simulink model "Model2_2023b"  (R2023b)
settings: Solver=ode4  StartTime=0.0  StopTime=100  FixedStep=0.01  RelTol=1e-3
values from neighbouring files (symbols this model uses):
  ARM_P_PID = [10 0 20]*0.1    [Single_ARM_Monte.m]    (also in main_starter.m)
  ARM_T_PID = [100 0 0]    [Single_ARM_Monte.m]    (also in main_starter.m)
  ARM_V_PID = [10 0 5]*0.1    [Single_ARM_Monte.m]    (also in main_starter.m)
  D_Joint0_angle0 = 45    [Single_ARM_Monte.m]    (also in main_starter.m)
  D_Joint0_angle1 = 0    [Single_ARM_Monte.m]    (also in main_starter.m)
  D_Joint0_angle2 = 0    [Single_ARM_Monte.m]    (also in main_starter.m)
  D_Joint0_rate0 = 0    [Single_ARM_Monte.m]    (also in main_starter.m)
  D_Joint0_rate1 = 0    [Single_ARM_Monte.m]    (also in main_starter.m)
  D_Joint0_rate2 = 0    [Single_ARM_Monte.m]    (also in main_starter.m)
  Joint_Motor_Mass = 23    [Single_ARM_Monte.m]    (also in main_starter.m)
  L_Joint0_angle0 = 45    [Single_ARM_Monte.m]    (also in main_starter.m)
  L_Joint0_angle1 = 0    [Single_ARM_Monte.m]    (also in main_starter.m)
  L_Joint0_angle2 = 0    [Single_ARM_Monte.m]    (also in main_starter.m)
  L_Joint0_rate0 = 0    [Single_ARM_Monte.m]    (also in main_starter.m)
  L_Joint0_rate1 = 0    [Single_ARM_Monte.m]    (also in main_starter.m)
  L_Joint0_rate2 = 0    [Single_ARM_Monte.m]    (also in main_starter.m)
  L_Joint_Offset = [ ... (first row only)    [Single_ARM_Monte.m]    (also in main_starter.m)
  Link1_Mass = 11    [Single_ARM_Monte.m]    (also in main_starter.m)
  Link2_Mass = 15.6    [Single_ARM_Monte.m]    (also in main_starter.m)
  Link3_Mass = 11    [Single_ARM_Monte.m]    (also in main_starter.m)
  Motor_transfer_Den = [1 100]    [Single_ARM_Monte.m]    (also in main_starter.m)
  Motor_transfer_Num = [100]    [Single_ARM_Monte.m]    (also in main_starter.m)
  PID_dt = 0.01    [Single_ARM_Monte.m]    (also in main_starter.m)
  R_Joint0_angle0 = 45    [Single_ARM_Monte.m]    (also in main_starter.m)
  R_Joint0_angle1 = 0    [Single_ARM_Monte.m]    (also in main_starter.m)
  R_Joint0_angle2 = 0    [Single_ARM_Monte.m]    (also in main_starter.m)
  R_Joint0_rate0 = 0    [Single_ARM_Monte.m]    (also in main_starter.m)
  R_Joint0_rate1 = 0    [Single_ARM_Monte.m]    (also in main_starter.m)
  R_Joint0_rate2 = 0    [Single_ARM_Monte.m]    (also in main_starter.m)
  RW_Att_D = 0.5    [Single_ARM_Monte.m]    (also in main_starter.m)
  RW_Att_I = 0.2    [Single_ARM_Monte.m]    (also in main_starter.m)
  RW_Att_P = 0.1    [Single_ARM_Monte.m]    (also in main_starter.m)
  RW_Mass = 100    [Single_ARM_Monte.m]    (also in main_starter.m)
  S_Body_Mass = 5    [Single_ARM_Monte.m]    (also in main_starter.m)
  S_init_pos = [0 0 0]'    [Single_ARM_Monte.m]    (also in main_starter.m)
  S_init_vel = [0 0 0]'    [Single_ARM_Monte.m]    (also in main_starter.m)
  T_Body_Mass = 4    [Single_ARM_Monte.m]    (also in main_starter.m)
  T_init_pos = [T_init_pos_list(i,1) T_init_pos_list(i,2) 0]'    [Single_ARM_Monte.m]    (also in main_starter.m = [1 0 0]')
  T_init_vel = [0 0 0]'    [Single_ARM_Monte.m]    (also in main_starter.m)
  Torq_mea_transfer_Den = [1 5]    [Single_ARM_Monte.m]    (also in main_starter.m)
  Torq_mea_transfer_Num = [5]    [Single_ARM_Monte.m]    (also in main_starter.m)
  U_Joint0_angle0 = 45    [Single_ARM_Monte.m]    (also in main_starter.m)
  U_Joint0_angle1 = 0    [Single_ARM_Monte.m]    (also in main_starter.m)
  U_Joint0_angle2 = 0    [Single_ARM_Monte.m]    (also in main_starter.m)
  U_Joint0_rate0 = 0    [Single_ARM_Monte.m]    (also in main_starter.m)
  U_Joint0_rate1 = 0    [Single_ARM_Monte.m]    (also in main_starter.m)
  U_Joint0_rate2 = 0    [Single_ARM_Monte.m]    (also in main_starter.m)
undefined symbols (not defined in the file or in its folder): X, Y, Z
libraries: nesl_utility x315, sm_lib x282, simulink_extras x46, sharedtransform x25, aerolibutil x4, simulink x2, matrix_library x2, dspmtrx3 x1
(part 1 of 12)
settings Model: Creator=yhj2019  LastModifiedBy=uscl
settings ExplorerConfigSet: InternalSimMechanicsExplorerSettings="<ExplorerConfiguration><canonicalview>default</canonicalview><AnimationSetting><BasePlaybackSpeed>1.0</BasePlaybackSpeed><PlaybackSpeedFactor>1.0</PlaybackSpeedFactor></AnimationSetting><TilePanel><TileInfo><Tiles Columns=\"1\" Count=\"1\" Rows=\"1\"><Column Weight=\"1\"/><Row Weight=\"1\"/><Tile Height=\"1\" Width=\"1\" X=\"0\" Y=\"0\"/></Tiles></TileInfo><SceneInfo><SceneViewer><BGColor><R>1</R><G>1</G><B>1</B></BGColor><Camera><DoPerspective>off</DoPerspective><Position><X>0.13582852589406158</X><Y>0.0815359438413352511</Y><Z>11.3316555905426526</Z></Position><Center><X>0.13582852589406158</X><Y>0.0815359438413352511</Y><Z>-0.00499986008405706173</Z></Center><Up><X>0</X><Y>1</Y><Z>-0</Z></Up><ViewLimDist>1</ViewLimDist><YLim>0.485687177104648538</YLim><XLim>0.453052070342676139</XLim></Camera></SceneViewer></SceneInfo></TilePanel><MechEditorPanel><Cameras/><GfxPanelCameraMap/><VideoCreator><PlaybackSpeedRatio>1.0</PlaybackSpeedRatio><FrameRate>30</FrameRate><VideoFormat>Motion JPEG AVI</VideoFormat><FrameSize>auto</FrameSize></VideoCreator></MechEditorPanel></ExplorerConfiguration>"

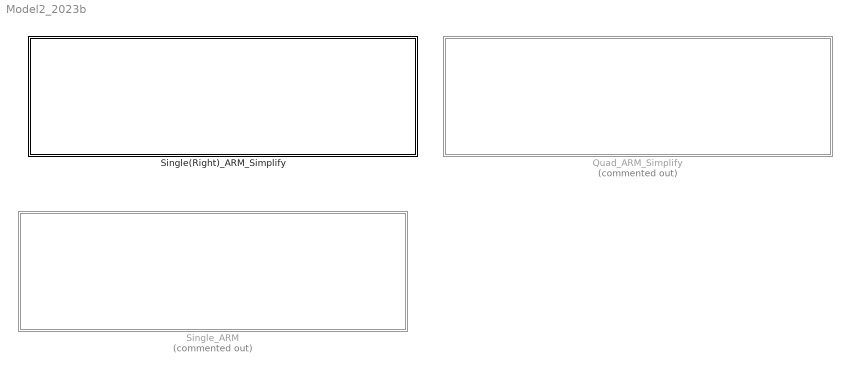
== system Model2_2023b ==
  Quad_ARM_Simplify : Subsystem  Commented=on
  Single(Right)_ARM_Simplify : Subsystem
  Single_ARM : Subsystem  Commented=on

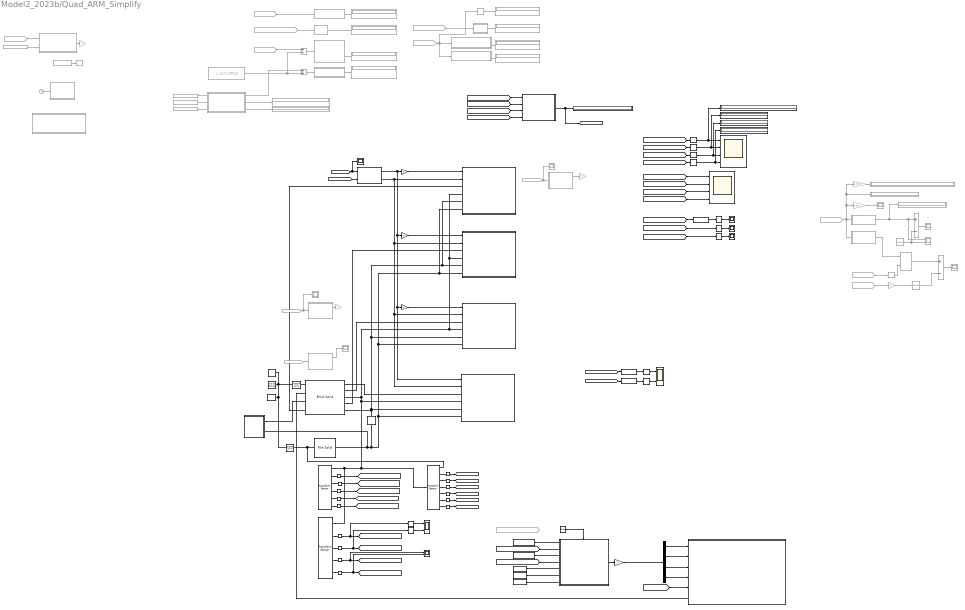
== system Model2_2023b/Quad_ARM_Simplify ==
  6-DOF Joint1 : sm_lib/Joints/6-DOF Joint  JointMode=Normal  CompositeWrenchDir=FollowerOnBase  CompositeWrenchFrame=BaseFrame  SenseConstraintForce=off  SenseConstraintTorque=off  SenseTotalForce=off  SenseTotalTorque=off  PxPositionTargetSpecify=on  PxPositionTargetPriority=High  PxPositionTargetValue=T_init_pos(1)  PxPositionTargetValueUnits=m  PxVelocityTargetSpecify=on  PxVelocityTargetPriority=High  PxVelocityTargetValue=T_init_vel(1)  PxVelocityTargetValueUnits=m/s  PxEquilibriumPosition=0  PxEquilibriumPositionUnits=m  PxSpringStiffness=0  PxSpringStiffnessUnits=N/m  PxDampingCoefficient=0  PxDampingCoefficientUnits=N/(m/s)  PxLowerLimitSpecify=off  PxLowerLimitBound=-1  PxLowerLimitBoundUnits=m  PxLowerLimitStiffness=1e6  PxLowerLimitStiffnessUnits=N/m  PxLowerLimitDamping=1e3  PxLowerLimitDampingUnits=N/(m/s)  PxLowerLimitTransitionRegionWidth=1e-4  PxLowerLimitTransitionRegionWidthUnits=m  PxUpperLimitSpecify=off  PxUpperLimitBound=1  PxUpperLimitBoundUnits=m  PxUpperLimitStiffness=1e6  PxUpperLimitStiffnessUnits=N/m  PxUpperLimitDamping=1e3  PxUpperLimitDampingUnits=N/(m/s)  PxUpperLimitTransitionRegionWidth=1e-4  PxUpperLimitTransitionRegionWidthUnits=m  PxTorqueActuationMode=NoTorque  PxMotionActuationMode=ComputedMotion  PxSensePosition=off  PxSenseVelocity=off  PxSenseAcceleration=off  PxSenseTorqueForce=off  PxSenseLowerLimitTorqueForce=off  PxSenseUpperLimitTorqueForce=off  PyPositionTargetSpecify=on  PyPositionTargetPriority=High  PyPositionTargetValue=T_init_pos(2)  PyPositionTargetValueUnits=m  PyVelocityTargetSpecify=on  PyVelocityTargetPriority=High  PyVelocityTargetValue=T_init_vel(2)  PyVelocityTargetValueUnits=m/s  PyEquilibriumPosition=0  PyEquilibriumPositionUnits=m  PySpringStiffness=0  PySpringStiffnessUnits=N/m  PyDampingCoefficient=0  PyDampingCoefficientUnits=N/(m/s)  PyLowerLimitSpecify=off  PyLowerLimitBound=-1  PyLowerLimitBoundUnits=m  PyLowerLimitStiffness=1e6  PyLowerLimitStiffnessUnits=N/m  PyLowerLimitDamping=1e3  PyLowerLimitDampingUnits=N/(m/s)  PyLowerLimitTransitionRegionWidth=1e-4  PyLowerLimitTransitionRegionWidthUnits=m  PyUpperLimitSpecify=off  PyUpperLimitBound=1  PyUpperLimitBoundUnits=m  PyUpperLimitStiffness=1e6  PyUpperLimitStiffnessUnits=N/m  PyUpperLimitDamping=1e3  PyUpperLimitDampingUnits=N/(m/s)  PyUpperLimitTransitionRegionWidth=1e-4  PyUpperLimitTransitionRegionWidthUnits=m  PyTorqueActuationMode=NoTorque  PyMotionActuationMode=ComputedMotion  PySensePosition=off  PySenseVelocity=off  PySenseAcceleration=off  PySenseTorqueForce=off  PySenseLowerLimitTorqueForce=off  PySenseUpperLimitTorqueForce=off  PzPositionTargetSpecify=on  PzPositionTargetPriority=High  PzPositionTargetValue=T_init_pos(3)  PzPositionTargetValueUnits=m  PzVelocityTargetSpecify=on  PzVelocityTargetPriority=High  PzVelocityTargetValue=T_init_vel(3)  PzVelocityTargetValueUnits=m/s  PzEquilibriumPosition=0  PzEquilibriumPositionUnits=m  PzSpringStiffness=0  PzSpringStiffnessUnits=N/m  PzDampingCoefficient=0  PzDampingCoefficientUnits=N/(m/s)  PzLowerLimitSpecify=off  PzLowerLimitBound=-1  PzLowerLimitBoundUnits=m  PzLowerLimitStiffness=1e6  PzLowerLimitStiffnessUnits=N/m  PzLowerLimitDamping=1e3  PzLowerLimitDampingUnits=N/(m/s)  PzLowerLimitTransitionRegionWidth=1e-4  PzLowerLimitTransitionRegionWidthUnits=m  PzUpperLimitSpecify=off  PzUpperLimitBound=1  PzUpperLimitBoundUnits=m  PzUpperLimitStiffness=1e6  PzUpperLimitStiffnessUnits=N/m  PzUpperLimitDamping=1e3  PzUpperLimitDampingUnits=N/(m/s)  PzUpperLimitTransitionRegionWidth=1e-4  PzUpperLimitTransitionRegionWidthUnits=m  PzTorqueActuationMode=NoTorque  PzMotionActuationMode=ComputedMotion  PzSensePosition=off  PzSenseVelocity=off  PzSenseAcceleration=off  PzSenseTorqueForce=off  PzSenseLowerLimitTorqueForce=off  PzSenseUpperLimitTorqueForce=off  SphPositionTargetSpecify=on  SphPositionTargetPriority=High  SphPositionTargetRotationMethod=RotationSequence  SphPositionTargetFollAlignAxisA=+X  SphPositionTargetBaseAlignAxisA=+Y  SphPositionTargetFollAlignAxisB=+Y  SphPositionTargetBaseAlignAxisB=+Z  SphPositionTargetRotationStandardAxis=+Z  SphPositionTargetRotationAngle=0.0  SphPositionTargetRotationAngleUnits=deg  SphPositionTargetRotationArbitraryAxis=[0 0 1]  SphPositionTargetRotationSequenceAxes=FollowerAxes  SphPositionTargetRotationSequence=ZYX  SphPositionTargetRotationSequenceAngles=T_init_att  SphPositionTargetRotationSequenceAnglesUnits=deg  SphPositionTargetRotationMatrix=[1 0 0; 0 1 0; 0 0 1]  SphPositionTargetQuaternion=[1 0 0 0]  SphVelocityTargetSpecify=on  SphVelocityTargetPriority=High  SphVelocityTargetValue=T_init_rate  SphVelocityTargetValueUnits=deg/s  SphVelocityTargetInFollowerFrame=on  SphEqPosRotationMethod=None  SphEqPosFollAlignAxisA=+X  SphEqPosBaseAlignAxisA=+Y  SphEqPosFollAlignAxisB=+Y  SphEqPosBaseAlignAxisB=+Z  SphEqPosRotationStandardAxis=+Z  SphEqPosRotationAngle=0.0  SphEqPosRotationAngleUnits=deg  SphEqPosRotationArbitraryAxis=[0 0 1]  SphEqPosRotationSequenceAxes=FollowerAxes  SphEqPosRotationSequence=XYX  SphEqPosRotationSequenceAngles=[0 0 0]  SphEqPosRotationSequenceAnglesUnits=deg  SphEqPosRotationMatrix=[1 0 0; 0 1 0; 0 0 1]  SphEqPosQuaternion=[1 0 0 0]  SphSpringStiffness=0  SphSpringStiffnessUnits=N*m/deg  SphDampingCoefficient=0  SphDampingCoefficientUnits=N*m/(deg/s)  SphLowerLimitSpecify=off  SphLowerLimitBound=15  SphLowerLimitBoundUnits=deg  SphLowerLimitStiffness=1e4  SphLowerLimitStiffnessUnits=N*m/deg  SphLowerLimitDamping=10  SphLowerLimitDampingUnits=N*m/(deg/s)  SphLowerLimitTransitionRegionWidth=0.1  SphLowerLimitTransitionRegionWidthUnits=deg  SphUpperLimitSpecify=off  SphUpperLimitBound=45  SphUpperLimitBoundUnits=deg  SphUpperLimitStiffness=1e4  SphUpperLimitStiffnessUnits=N*m/deg  SphUpperLimitDamping=10  SphUpperLimitDampingUnits=N*m/(deg/s)  SphUpperLimitTransitionRegionWidth=0.1  SphUpperLimitTransitionRegionWidthUnits=deg  SphTorqueActuationMode=NoTorque  SphActuateTorqueX=off  SphActuateTorqueY=off  SphActuateTorqueZ=off  SphActuateTorque=off  SphActuationFrame=BaseFrame  SphSensePosition=off  SphSenseVelocityX=off  SphSenseVelocityY=off  SphSenseVelocityZ=off  SphSenseVelocity=off  SphSenseAccelerationX=off  SphSenseAccelerationY=off  SphSenseAccelerationZ=off  SphSenseAcceleration=off  SphSenseLowerLimitTorqueMag=off  SphSenseUpperLimitTorqueMag=off  SphSensingFrame=BaseFrame
  6-DOF Joint2 : sm_lib/Joints/6-DOF Joint  JointMode=Normal  CompositeWrenchDir=FollowerOnBase  CompositeWrenchFrame=BaseFrame  SenseConstraintForce=off  SenseConstraintTorque=off  SenseTotalForce=off  SenseTotalTorque=off  PxPositionTargetSpecify=on  PxPositionTargetPriority=High  PxPositionTargetValue=S_init_pos(1)  PxPositionTargetValueUnits=m  PxVelocityTargetSpecify=on  PxVelocityTargetPriority=High  PxVelocityTargetValue=S_init_vel(1)  PxVelocityTargetValueUnits=m/s  PxEquilibriumPosition=0  PxEquilibriumPositionUnits=m  PxSpringStiffness=0  PxSpringStiffnessUnits=N/m  PxDampingCoefficient=0  PxDampingCoefficientUnits=N/(m/s)  PxLowerLimitSpecify=off  PxLowerLimitBound=-1  PxLowerLimitBoundUnits=m  PxLowerLimitStiffness=1e6  PxLowerLimitStiffnessUnits=N/m  PxLowerLimitDamping=1e3  PxLowerLimitDampingUnits=N/(m/s)  PxLowerLimitTransitionRegionWidth=1e-4  PxLowerLimitTransitionRegionWidthUnits=m  PxUpperLimitSpecify=off  PxUpperLimitBound=1  PxUpperLimitBoundUnits=m  PxUpperLimitStiffness=1e6  PxUpperLimitStiffnessUnits=N/m  PxUpperLimitDamping=1e3  PxUpperLimitDampingUnits=N/(m/s)  PxUpperLimitTransitionRegionWidth=1e-4  PxUpperLimitTransitionRegionWidthUnits=m  PxTorqueActuationMode=NoTorque  PxMotionActuationMode=ComputedMotion  PxSensePosition=off  PxSenseVelocity=off  PxSenseAcceleration=off  PxSenseTorqueForce=off  PxSenseLowerLimitTorqueForce=off  PxSenseUpperLimitTorqueForce=off  PyPositionTargetSpecify=on  PyPositionTargetPriority=High  PyPositionTargetValue=S_init_pos(2)  PyPositionTargetValueUnits=m  PyVelocityTargetSpecify=on  PyVelocityTargetPriority=High  PyVelocityTargetValue=S_init_vel(2)  PyVelocityTargetValueUnits=m/s  PyEquilibriumPosition=0  PyEquilibriumPositionUnits=m  PySpringStiffness=0  PySpringStiffnessUnits=N/m  PyDampingCoefficient=0  PyDampingCoefficientUnits=N/(m/s)  PyLowerLimitSpecify=off  PyLowerLimitBound=-1  PyLowerLimitBoundUnits=m  PyLowerLimitStiffness=1e6  PyLowerLimitStiffnessUnits=N/m  PyLowerLimitDamping=1e3  PyLowerLimitDampingUnits=N/(m/s)  PyLowerLimitTransitionRegionWidth=1e-4  PyLowerLimitTransitionRegionWidthUnits=m  PyUpperLimitSpecify=off  PyUpperLimitBound=1  PyUpperLimitBoundUnits=m  PyUpperLimitStiffness=1e6  PyUpperLimitStiffnessUnits=N/m  PyUpperLimitDamping=1e3  PyUpperLimitDampingUnits=N/(m/s)  PyUpperLimitTransitionRegionWidth=1e-4  PyUpperLimitTransitionRegionWidthUnits=m  PyTorqueActuationMode=NoTorque  PyMotionActuationMode=ComputedMotion  PySensePosition=off  PySenseVelocity=off  PySenseAcceleration=off  PySenseTorqueForce=off  PySenseLowerLimitTorqueForce=off  PySenseUpperLimitTorqueForce=off  PzPositionTargetSpecify=on  PzPositionTargetPriority=High  PzPositionTargetValue=S_init_pos(3)  PzPositionTargetValueUnits=m  PzVelocityTargetSpecify=on  PzVelocityTargetPriority=High  PzVelocityTargetValue=S_init_vel(3)  PzVelocityTargetValueUnits=m/s  PzEquilibriumPosition=0  PzEquilibriumPositionUnits=m  PzSpringStiffness=0  PzSpringStiffnessUnits=N/m  PzDampingCoefficient=0  PzDampingCoefficientUnits=N/(m/s)  PzLowerLimitSpecify=off  PzLowerLimitBound=-1  PzLowerLimitBoundUnits=m  PzLowerLimitStiffness=1e6  PzLowerLimitStiffnessUnits=N/m  PzLowerLimitDamping=1e3  PzLowerLimitDampingUnits=N/(m/s)  PzLowerLimitTransitionRegionWidth=1e-4  PzLowerLimitTransitionRegionWidthUnits=m  PzUpperLimitSpecify=off  PzUpperLimitBound=1  PzUpperLimitBoundUnits=m  PzUpperLimitStiffness=1e6  PzUpperLimitStiffnessUnits=N/m  PzUpperLimitDamping=1e3  PzUpperLimitDampingUnits=N/(m/s)  PzUpperLimitTransitionRegionWidth=1e-4  PzUpperLimitTransitionRegionWidthUnits=m  PzTorqueActuationMode=NoTorque  PzMotionActuationMode=ComputedMotion  PzSensePosition=off  PzSenseVelocity=off  PzSenseAcceleration=off  PzSenseTorqueForce=off  PzSenseLowerLimitTorqueForce=off  PzSenseUpperLimitTorqueForce=off  SphPositionTargetSpecify=on  SphPositionTargetPriority=High  SphPositionTargetRotationMethod=RotationSequence  SphPositionTargetFollAlignAxisA=+X  SphPositionTargetBaseAlignAxisA=+Y  SphPositionTargetFollAlignAxisB=+Y  SphPositionTargetBaseAlignAxisB=+Z  SphPositionTargetRotationStandardAxis=+Z  SphPositionTargetRotationAngle=0.0  SphPositionTargetRotationAngleUnits=deg  SphPositionTargetRotationArbitraryAxis=[0 0 1]  SphPositionTargetRotationSequenceAxes=FollowerAxes  SphPositionTargetRotationSequence=ZYX  SphPositionTargetRotationSequenceAngles=S_init_att  SphPositionTargetRotationSequenceAnglesUnits=deg  SphPositionTargetRotationMatrix=[1 0 0; 0 1 0; 0 0 1]  SphPositionTargetQuaternion=[1 0 0 0]  SphVelocityTargetSpecify=on  SphVelocityTargetPriority=High  SphVelocityTargetValue=S_init_rate  SphVelocityTargetValueUnits=deg/s  SphVelocityTargetInFollowerFrame=on  SphEqPosRotationMethod=None  SphEqPosFollAlignAxisA=+X  SphEqPosBaseAlignAxisA=+Y  SphEqPosFollAlignAxisB=+Y  SphEqPosBaseAlignAxisB=+Z  SphEqPosRotationStandardAxis=+Z  SphEqPosRotationAngle=0.0  SphEqPosRotationAngleUnits=deg  SphEqPosRotationArbitraryAxis=[0 0 1]  SphEqPosRotationSequenceAxes=FollowerAxes  SphEqPosRotationSequence=XYX  SphEqPosRotationSequenceAngles=[0 0 0]  SphEqPosRotationSequenceAnglesUnits=deg  SphEqPosRotationMatrix=[1 0 0; 0 1 0; 0 0 1]  SphEqPosQuaternion=[1 0 0 0]  SphSpringStiffness=0  SphSpringStiffnessUnits=N*m/deg  SphDampingCoefficient=0  SphDampingCoefficientUnits=N*m/(deg/s)  SphLowerLimitSpecify=off  SphLowerLimitBound=15  SphLowerLimitBoundUnits=deg  SphLowerLimitStiffness=1e4  SphLowerLimitStiffnessUnits=N*m/deg  SphLowerLimitDamping=10  SphLowerLimitDampingUnits=N*m/(deg/s)  SphLowerLimitTransitionRegionWidth=0.1  SphLowerLimitTransitionRegionWidthUnits=deg  SphUpperLimitSpecify=off  SphUpperLimitBound=45  SphUpperLimitBoundUnits=deg  SphUpperLimitStiffness=1e4  SphUpperLimitStiffnessUnits=N*m/deg  SphUpperLimitDamping=10  SphUpperLimitDampingUnits=N*m/(deg/s)  SphUpperLimitTransitionRegionWidth=0.1  SphUpperLimitTransitionRegionWidthUnits=deg  SphTorqueActuationMode=NoTorque  SphActuateTorqueX=off  SphActuateTorqueY=off  SphActuateTorqueZ=off  SphActuateTorque=off  SphActuationFrame=BaseFrame  SphSensePosition=off  SphSenseVelocityX=off  SphSenseVelocityY=off  SphSenseVelocityZ=off  SphSenseVelocity=off  SphSenseAccelerationX=off  SphSenseAccelerationY=off  SphSenseAccelerationZ=off  SphSenseAcceleration=off  SphSenseLowerLimitTorqueMag=off  SphSenseUpperLimitTorqueMag=off  SphSensingFrame=BaseFrame
  Add1 : Sum  Commented=on  Inputs=+-
  Add2 : Sum  Commented=on  Inputs=+-
  Add3 : Sum  Commented=on
  Add5 : Sum  Commented=on  Inputs=+-
  Attitude:Rel,Iner : Scope  NumInputPorts=2
  Brick Solid : sm_lib/Body Elements/Brick Solid  BrickDimensions=[30 30 40]  BrickDimensionsUnits=cm  ExportEntireGeometry=on  InertiaType=CalculateFromGeometry  BasedOnType=Mass  Density=1000  DensityUnits=kg/m^3  Mass=S_Body_Mass  MassUnits=kg  CenterOfMass=[0 0 0]  CenterOfMassUnits=m  MomentsOfInertia=[1 1 1]  MomentsOfInertiaUnits=kg*m^2  ProductsOfInertia=[0 0 0]  ProductsOfInertiaUnits=kg*m^2  GraphicType=FromGeometry  MarkerShape=Sphere  MarkerSize=10  GraphicVisPropType=SimpleVisualProperties  GraphicDiffuseColor=[0.4 0.4 0.4]  GraphicOpacity=0.2  GraphicSpecularColor=[0.5 0.5 0.5 1.0]  GraphicAmbientColor=[0.15 0.15 0.15 1.0]  GraphicEmissiveColor=[0.0 0.0 0.0 1.0]  GraphicShininess=75  DoExposeReferenceFrame=on  SerializedFrames=<Frames><Frame><Id>Frame1</Id><Value><Name>Left_AMR_F</Name><Origin><Source>CenterOfMassFrame</Source><FeatureName></FeatureName></Origin><PrimaryAxis><DefinedDirection>+Z</DefinedDirection><Source>ReferenceFrame</Source><SourceDirection>+Z</SourceDirection><FeatureName></FeatureName></PrimaryAxis><SecondaryAxis><DefinedDirection>+X</DefinedDirection><Source>ReferenceFrame</Source><SourceDirection>+X</SourceDirection><FeatureName></FeatureName></SecondaryAxis></Value></Frame><Frame><Id>Frame2</Id><Value><Name>Right_ARM_F</Name><Origin><Source>ReferenceFrame</Source><FeatureName></FeatureName></Origin><PrimaryAxis><DefinedDirection>+Z</DefinedDirection><Source>ReferenceFrame</Source><SourceDirection>+Z</SourceDirection><FeatureName></FeatureName></PrimaryAxis><SecondaryAxis><DefinedDirection>+X</DefinedDirection><Source>ReferenceFrame</Source><SourceDirection>+X</SourceDirection><FeatureName></FeatureName></SecondaryAxis></Value></Frame><Frame><Id>Frame3</Id><Value><Name>RW_F</Name><Origin><Source>CenterOfMassFrame</Source><FeatureName></FeatureName></Origin><PrimaryAxis><DefinedDirection>+Z</DefinedDirection><Source>ReferenceFrame</Source><SourceDirection>+Z</SourceDirection><FeatureName></FeatureName></PrimaryAxis><SecondaryAxis><DefinedDirection>+X</DefinedDirection><Source>ReferenceFrame</Source><SourceDirection>+X</SourceDirection><FeatureName></FeatureName></SecondaryAxis></Value></Frame><Frame><Id>Frame4</Id><Value><Name>CoM_F</Name><Origin><Source>ReferenceFrame</Source><FeatureName></FeatureName></Origin><PrimaryAxis><DefinedDirection>+Z</DefinedDirection><Source>ReferenceFrame</Source><SourceDirection>+Z</SourceDirection><FeatureName></FeatureName></PrimaryAxis><SecondaryAxis><DefinedDirection>+X</DefinedDirection><Source>ReferenceFrame</Source><SourceDirection>+X</SourceDirection><FeatureName></FeatureName></SecondaryAxis></Value></Frame><Frame><Id>Frame5</Id><Value><Name>Body_Contact_Sensor_F</Name><Origin><Source>GeometricFeature</Source><FeatureName>+x surface</FeatureName></Origin><PrimaryAxis><DefinedDirection>+Z</DefinedDirection><Source>ReferenceFrame</Source><SourceDirection>+Z</SourceDirection><FeatureName></FeatureName></PrimaryAxis><SecondaryAxis><DefinedDirection>+X</DefinedDirection><Source>ReferenceFrame</Source><SourceDirection>+X</SourceDirection><FeatureName></FeatureName></SecondaryAxis></Value></Frame><Frame><Id>Frame6</Id><Value><Name>Up_ARM_F</Name><Origin><Source>ReferenceFrame</Source><FeatureName></FeatureName></Origin><PrimaryAxis><DefinedDirection>+Z</DefinedDirection><Source>ReferenceFrame</Source><SourceDirection>+Z</SourceDirection><FeatureName></FeatureName></PrimaryAxis><SecondaryAxis><DefinedDirection>+X</DefinedDirection><Source>ReferenceFrame</Source><SourceDirection>+X</SourceDirection><FeatureName></FeatureName></SecondaryAxis></Value></Frame><Frame><Id>Frame7</Id><Value><Name>Down_ARM_F</Name><Origin><Source>ReferenceFrame</Source><FeatureName></FeatureName></Origin><PrimaryAxis><DefinedDirection>+Z</DefinedDirection><Source>ReferenceFrame</Source><SourceDirection>+Z</SourceDirection><FeatureName></FeatureName></PrimaryAxis><SecondaryAxis><DefinedDirection>+X</DefinedDirection><Source>ReferenceFrame</Source><SourceDirection>+X</SourceDirection><FeatureName></FeatureName></SecondaryAxis></Value></Frame></Frames>
  Clock1 : Clock  Commented=on
  Constant : Constant  Commented=on  Value=L_Joint_Offset
  Constant1 : Constant  Value=[0 0 0]'
  Constant10 : Constant  Value=RW_Att_D
  Constant2 : Constant  Commented=on  Value=[0.3 0.3]'
  Constant3 : Constant  Commented=on  Value=[0.3 0.3]'
  Constant4 : Constant  Commented=on  Value=0.001
  Constant5 : Constant  Commented=on  Value=100
  Constant6 : Constant  Commented=on  Value=[45 -90 -180]'
  Constant7 : Constant  Value=[0 0 0]'
  Constant8 : Constant  Value=RW_Att_P
  Constant9 : Constant  Value=RW_Att_I
  Degrees to Radians : simulink_extras/Transformations/Degrees to Radians  Commented=on
  Demux1 : Demux
  Display{,1..8,14..17} (13 alike) : Display  Commented=on
  Display{9..13} (5 alike) : Display
  Down_ARM : Subsystem
  End_Position_Flg : MATLAB Function  TreatAsAtomicUnit=on
  Fabrik_based_EE_Control(Angle) : MATLAB Function  Commented=on  TreatAsAtomicUnit=on
  From1 : From  Commented=on  GotoTag=LEFT_ARM_J  TagVisibility=global
  From12 : From  Commented=on  GotoTag=LEFT_ARM_J  TagVisibility=global
  From13 : From  Commented=on  GotoTag=B_f_contact  TagVisibility=global
  From14 : From  Commented=on  GotoTag=LEFT_ARM_Jd  TagVisibility=global
  From16 : From  Commented=on  GotoTag=Relative_quat
  From19 : From  Commented=on  GotoTag=B_f_contact  TagVisibility=global
  From2 : From  Commented=on  GotoTag=ARM_J  TagVisibility=global
  From24 : From  Commented=on  GotoTag=LEFT_EE_Vel
  From3 : From  Commented=on  GotoTag=LEFT_ARM_J_Pos_Mount  TagVisibility=global
  From33 : From  Commented=on  GotoTag=Right_ARM_J  TagVisibility=global
  From34 : From  Commented=on  GotoTag=Right_ARM_J_Pos_Mount  TagVisibility=global
  From4 : From  Commented=on  GotoTag=LEFT_ARM_J  TagVisibility=global
  From9 : From  Commented=on  GotoTag=B_f_contact  TagVisibility=global
  Gain : Gain  Commented=on
  Gain1 : Gain  Commented=on  Gain=-1
  Gain2 : Gain
  Gain3 : Gain  Commented=on
  Gain4 : Gain  Commented=on  Gain=180/pi
  Gain5 : Gain  Commented=on  Gain=-1
  Gain6 : Gain  Commented=on  Gain=180/pi
  Gain7 : Gain
  Gain8 : Gain  Gain=-1
  Gain9 : Gain  Gain=-1
  Jacobian_based_EE_Control(Rate) : MATLAB Function  Commented=on  TreatAsAtomicUnit=on
  Joint_Angle_Mea:LEFT,Right,Down,Up : Scope  NumInputPorts=4
  Left_ARM : Subsystem
  MATLAB Function : MATLAB Function  Commented=on  TreatAsAtomicUnit=on
  MATLAB Function1 : MATLAB Function  Commented=on  TreatAsAtomicUnit=on
  MATLAB Function2 : MATLAB Function  Commented=on  TreatAsAtomicUnit=on
  MATLAB Function3 : MATLAB Function  Commented=on  TreatAsAtomicUnit=on
  MATLAB Function4 : MATLAB Function  Commented=on  TreatAsAtomicUnit=on
  MATLAB Function5 : MATLAB Function  Commented=on  TreatAsAtomicUnit=on
  MATLAB Function6 : MATLAB Function  Commented=on  TreatAsAtomicUnit=on
  Matrix Multiply : Product  Commented=on  Multiplication=Matrix(*)
  Mechanism Configuration : sm_lib/Utilities/Mechanism Configuration  UniformGravity=None  GravityVector=[0 0 -9.80665]  GravityVectorUnits=m/s^2  LinearizationDelta=0.001  JointModeTransitionNonlinearIterations=2
  Mount_Frame_Based_Jacobian_Test : Subsystem  Commented=on
  Openning_Motion_Sequence : MATLAB Function  Commented=on  TreatAsAtomicUnit=on
  Openning_Motion_Sequence1 : MATLAB Function  Commented=on  TreatAsAtomicUnit=on
  Openning_Motion_Sequence2 : MATLAB Function  Commented=on  TreatAsAtomicUnit=on
  Openning_Motion_Sequence3 : MATLAB Function  Commented=on  TreatAsAtomicUnit=on
  Openning_Motion_Sequence4 : MATLAB Function  TreatAsAtomicUnit=on
  PS-Simulink Converter{1..7,13..15,23,26..28,38} (15 alike) : nesl_utility/PS-Simulink Converter  PhysicalDomain=network_engine_domain  SubClassName=ps_output  LeftPortType=input  RightPortType=output  PseudoPeriodic=off  Frequencies=[]  VectorFormat=inherit  Unit=inherit  AffineConversion=off
  Pulse Generator : DiscretePulseGenerator  PulseType=Time based  Period=0.2  PulseWidth=50
  Quaternions to Rotation Angles : sharedtransform/Quaternions to Rotation Angles  rotationOrder=ZYX  aMode=aMode
  Quaternions to Rotation Angles1 : sharedtransform/Quaternions to Rotation Angles  rotationOrder=ZYX  aMode=aMode
  Quaternions to Rotation Angles2 : sharedtransform/Quaternions to Rotation Angles  rotationOrder=ZYX  aMode=aMode
  Radians to Degrees{,1..10} (11 alike) : simulink_extras/Transformations/Radians to Degrees
  Radians to Degrees11 : simulink_extras/Transformations/Radians to Degrees  Commented=on
  Reshape7 : Reshape  Commented=on  OutputDimensionality=Column vector (2-D)
  Right_ARM : Subsystem
  Right_ARM_Real_FK : MATLAB Function  Commented=on  TreatAsAtomicUnit=on
  Right_ARM_Real_Simple_FK : MATLAB Function  Commented=on  TreatAsAtomicUnit=on
  Scope{,1,3,11..12,15} (6 alike) : Scope  Commented=on
  Scope{4,6,8,16} (4 alike) : Scope
  Scope2 : Scope  Commented=on  NumInputPorts=2
  Scope5 : Scope  NumInputPorts=2
  Scope7 : Scope  NumInputPorts=2
  Selector1 : Selector  Commented=on  InputPortWidth=3  IndexOptions=Index vector (dialog)  Indices=[1 2]  OutputSizes=1
  Selector2 : Selector  Commented=on  InputPortWidth=3  IndexOptions=Index vector (dialog)  Indices=[1 2]  OutputSizes=1
  Solver Configuration : nesl_utility/Solver Configuration  PhysicalDomain=network_engine_domain  SubClassName=solver  LeftPortType=input  RightPortType=generic  Tones=[]  Harmonics=[]  SimulateNoise=off  Profile=off  UseLocalSampling=off  EnableSwitchedLinearOptims=on  FrequencyDomain=off  UseCCode=off  RelTol=0.001  AbsTol=0.001  MinStep=1e-09  ToWorkspace=off  RevertToSquareIcSolve=off  NumHomotopyIterations=100  PhasorMode=off  PhasorModeNumHarmonics=1  ConsistencySolver=NEWTON_XTOL_AFTER_FTOL  IndexReductionMethod=DerivativeReplacement  DoDC=off  ResidualTolerance=1e-09  ConsistencyTolSource=GLOBAL  ConsistencyAbsTol=0.001  ConsistencyRelTol=0.001  ConsistencyTolFactor=0.001  UseLocalSolver=off  LocalSolverChoice=NE_BACKWARD_EULER_ADVANCER  ResolveIndetEquations=on  FunctionEvalNumThread=1  LocalSolverSampleTime=0.001  DoFixedCost=off  MaxNonlinIter=3  MaxModeIter=2  ComputeImpulses=off  ImpulseIterations=2  LinearAlgebra=auto  LinearAlgebraNumThread=0  EquationFormulation=NE_TIME_EF  DelaysMemoryBudget=1024  AutomaticFiltering=on  FilteringTimeConstant=0.001  PartitionStorageMethod=AS_NEEDED  PartitionMemoryBudget=1024  PartitionMethod=ROBUST  MultibodyUseLocalSolver=off  MultibodyLocalSolverChoice=ODE1  MultibodyLocalSolverSampleTime=0.001
  Spatial Contact Force6 : sm_lib/Forces and Torques/Spatial Contact Force  NormalForceType=SmoothSpringDamper  NormalStiffness=B2T_Siffness  NormalStiffnessUnits=N/m  NormalDamping=B2T_Damping  NormalDampingUnits=N/(m/s)  NormalTransitionRegionWidth=B2T_TRW  NormalTransitionRegionWidthUnits=m  FrictionType=SmoothStickSlip  CoefficientOfStaticFriction=0.8  CoefficientOfDynamicFriction=0.6  FrictionalCriticalVelocity=1e-3  FrictionalCriticalVelocityUnits=m/s  SenseContactSignal=off  SensePenetrationDepth=off  SenseSeparationDistance=off  SenseNormalForceMagnitude=off  SenseFrictionalForceMagnitude=off  SenseNormalVelocity=off  SenseTangentialVelocity=off  SenseContactBaseRotation=off  SenseContactBaseTranslation=off  SenseContactFollowerRotation=off  SenseContactFollowerTranslation=off  ZeroCrossDetectContactStartAndEnd=off
  Subsystem1 : Subsystem
  Subsystem2 : Subsystem
  Subsystem5 : Subsystem
  Target : sm_lib/Body Elements/File Solid  ExtGeomFileName=../\target_model\cubesat_12_0U.stl  UnitType=Custom  ExtGeomFileUnits=mm  StepReaderType=HEX  ExportConvexHullGeometry=on  InertiaType=CalculateFromGeometry  BasedOnType=Mass  Density=1000  DensityUnits=kg/m^3  Mass=T_Body_Mass  MassUnits=kg  CenterOfMass=[0 0 0]  CenterOfMassUnits=m  MomentsOfInertia=[1 1 1]  MomentsOfInertiaUnits=kg*m^2  ProductsOfInertia=[0 0 0]  ProductsOfInertiaUnits=kg*m^2  GraphicType=FromGeometry  MarkerShape=Sphere  MarkerSize=10  GraphicVisPropType=SimpleVisualProperties  GraphicDiffuseColor=[0.8 0.0 0.2]  GraphicOpacity=1  GraphicSpecularColor=[0.5 0.5 0.5 1.0]  GraphicAmbientColor=[0.15 0.15 0.15 1.0]  GraphicEmissiveColor=[0.0 0.0 0.0 1.0]  GraphicShininess=75  DoExposeReferenceFrame=on  SerializedFrames=<Frames/>
  Torq_Mea:LEFT,Right,Down,Up : Scope  NumInputPorts=4
  Transform Sensor1 : sm_lib/Frames and Transforms/Transform Sensor  MeasurementFrame=Follower  RotationSequence=ZYX  SenseAngle=off  SenseAxis=off  SenseQ=off  SenseR=off  SenseRotationSequence=off  SenseOmegaX=off  SenseOmegaY=off  SenseOmegaZ=off  SenseOmega=on  SenseQDot=off  SenseRDot=off  SenseRotationSequenceDot=off  SenseAlphaX=off  SenseAlphaY=off  SenseAlphaZ=off  SenseAlpha=on  SenseQDDot=off  SenseRDDot=off  SenseX=off  SenseY=off  SenseZ=off  SenseXYZ=off  SenseRad=off  SenseAzim=off  SenseDist=off  SenseInc=off  SenseXDot=off  SenseYDot=off  SenseZDot=off  SenseXYZDot=on  SenseRadDot=off  SenseAzimDot=off  SenseDistDot=off  SenseIncDot=off  SenseXDDot=off  SenseYDDot=off  SenseZDDot=off  SenseXYZDDot=on  SenseRadDDot=off  SenseAzimDDot=off  SenseDistDDot=off  SenseIncDDot=off
  Transform Sensor2 : sm_lib/Frames and Transforms/Transform Sensor  MeasurementFrame=Base  RotationSequence=ZYX  SenseAngle=off  SenseAxis=off  SenseQ=on  SenseR=off  SenseRotationSequence=off  SenseOmegaX=off  SenseOmegaY=off  SenseOmegaZ=off  SenseOmega=on  SenseQDot=off  SenseRDot=off  SenseRotationSequenceDot=off  SenseAlphaX=off  SenseAlphaY=off  SenseAlphaZ=off  SenseAlpha=on  SenseQDDot=off  SenseRDDot=off  SenseX=off  SenseY=off  SenseZ=off  SenseXYZ=on  SenseRad=off  SenseAzim=off  SenseDist=off  SenseInc=off  SenseXDot=off  SenseYDot=off  SenseZDot=off  SenseXYZDot=on  SenseRadDot=off  SenseAzimDot=off  SenseDistDot=off  SenseIncDot=off  SenseXDDot=off  SenseYDDot=off  SenseZDDot=off  SenseXYZDDot=on  SenseRadDDot=off  SenseAzimDDot=off  SenseDistDDot=off  SenseIncDDot=off
  Transform Sensor5 : sm_lib/Frames and Transforms/Transform Sensor  MeasurementFrame=World  RotationSequence=ZYX  SenseAngle=off  SenseAxis=off  SenseQ=on  SenseR=on  SenseRotationSequence=off  SenseOmegaX=off  SenseOmegaY=off  SenseOmegaZ=off  SenseOmega=off  SenseQDot=off  SenseRDot=off  SenseRotationSequenceDot=off  SenseAlphaX=off  SenseAlphaY=off  SenseAlphaZ=off  SenseAlpha=off  SenseQDDot=off  SenseRDDot=off  SenseX=off  SenseY=off  SenseZ=off  SenseXYZ=on  SenseRad=off  SenseAzim=off  SenseDist=off  SenseInc=off  SenseXDot=off  SenseYDot=off  SenseZDot=off  SenseXYZDot=on  SenseRadDot=off  SenseAzimDot=off  SenseDistDot=off  SenseIncDot=off  SenseXDDot=off  SenseYDDot=off  SenseZDDot=off  SenseXYZDDot=on  SenseRadDDot=off  SenseAzimDDot=off  SenseDistDDot=off  SenseIncDDot=off
  Up_ARM : Subsystem
  World Frame : sm_lib/Frames and Transforms/World Frame
  tag scope: S_Acc_wrt_Body=global, S_Acc_wrt_Inertial=global, S_Attitude_quat_Inertial=global, S_Pos_wrt_Inertial=global, S_Rate_wrt_Body=global, S_Rated_wrt_Body=global, S_Vel_wrt_Body=global, S_Vel_wrt_Inertial=global
  wires:
  MATLAB Function1/1(J) -> Matrix Multiply/1
  Selector1/1 -> Add1/2, Scope2/2
  From12/1 -> MATLAB Function/1(theta), Gain4/1, Display2/1, Gain6/1, MATLAB Function1/1(theta)
  From14/1 -> Reshape7/1
  Gain4/1 -> Scope/1
  MATLAB Function/1(pos) -> Display5/1, Scope2/1, Add1/1
  Radians to Degrees/1 -> Scope4/1
  Matrix Multiply/1 -> Add2/1
  Radians to Degrees2/1 -> Scope6/1
  Add1/1 -> Scope1/1
  Gain6/1 -> Display3/1
  From24/1 -> Gain3/1
  Selector2/1 -> Add2/2
  Gain3/1 -> Selector2/1
  Quaternions to Rotation Angles/1 -> Radians to Degrees/1
  Add2/1 -> Scope3/1
  Reshape7/1 -> Matrix Multiply/2
  From2/1 -> Jacobian_based_EE_Control(Rate)/1(q)
  Constant2/1 -> Jacobian_based_EE_Control(Rate)/2(target_pos)
  Constant3/1 -> Fabrik_based_EE_Control(Angle)/1(target)
  Fabrik_based_EE_Control(Angle)/1(q_list) -> Add3/1
  Fabrik_based_EE_Control(Angle)/2(pos_list) -> Display/1
  Jacobian_based_EE_Control(Rate)/1(qd_cmd) -> Gain/1
  Constant4/1 -> Fabrik_based_EE_Control(Angle)/2(tol)
  Constant5/1 -> Fabrik_based_EE_Control(Angle)/3(max_iter)
  MATLAB Function5/1(pos) -> Display1/1
  Fabrik_based_EE_Control(Angle)/3(iter_fin) -> Display6/1
  MATLAB Function6/2(ee_pose) -> Display7/1
  Add3/1 -> MATLAB Function5/1(theta)
  Constant/1 -> Add3/2, Add5/2
  From3/1 -> MATLAB Function2/1(u)
  Constant6/1 -> Degrees to Radians/1
  From13/1 -> Openning_Motion_Sequence/1(b_flg)
  MATLAB Function2/1(y) -> Display4/1
  From1/1 -> MATLAB Function3/1(theta)
  MATLAB Function3/1(pos) -> Display8/1
  Add5/1 -> MATLAB Function6/1(theta)
  From4/1 -> Add5/1
  PS-Simulink Converter23/1 -> [S_Attitude_quat_Inertial]
  PS-Simulink Converter26/1 -> [S_Pos_wrt_Inertial]
  PS-Simulink Converter27/1 -> [S_Vel_wrt_Inertial]
  PS-Simulink Converter28/1 -> [S_Acc_wrt_Inertial]
  PS-Simulink Converter2/1 -> Radians to Degrees3/1, [S_Rated_wrt_Body]
  PS-Simulink Converter1/1 -> Radians to Degrees1/1, [S_Rate_wrt_Body]
  PS-Simulink Converter3/1 -> Scope7/1, [S_Vel_wrt_Body]
  PS-Simulink Converter4/1 -> [S_Acc_wrt_Body], Scope7/2
  Radians to Degrees1/1 -> Scope5/1
  Radians to Degrees3/1 -> Scope5/2
  [S_Attitude_quat_Inertial] -> Quaternions to Rotation Angles/1
  [S_Rate_wrt_Body] -> Radians to Degrees2/1
  [S_Rated_wrt_Body] -> Radians to Degrees4/1
  Radians to Degrees4/1 -> Scope8/1
  Clock1/1 -> Openning_Motion_Sequence1/1(t)
  Openning_Motion_Sequence/1(res) -> Scope11/1
  Constant8/1 -> Subsystem1/5(P_gain)
  [S_Rate_wrt_Body] -> Subsystem1/4(In4)
  Constant9/1 -> Subsystem1/6(I_gain)
  Constant1/1 -> Subsystem1/1(Degrees in)
  Gain2/1 -> Demux1/1
  Subsystem1/1(Omegad) -> Gain2/1
  Pulse Generator/1 -> Subsystem1/Trigger
  Constant7/1 -> Subsystem1/3(In3)
  Constant10/1 -> Subsystem1/7(D_gain)
  PS-Simulink Converter38/1 -> [Service_Body_R]
  Demux1/1 -> Subsystem5/1(RW1_Torque_CMD)
  Demux1/2 -> Subsystem5/2(RW2_Torque_CMD)
  Demux1/3 -> Subsystem5/3(RW3_Torque_CMD)
  Demux1/4 -> Subsystem5/4(RW4_Torque_CMD)
  [Service_Body_R] -> Subsystem5/5(Satellite_Attitude)
  PS-Simulink Converter13/1 -> [Relative_pos]
  PS-Simulink Converter14/1 -> [Relative_Acc]
  PS-Simulink Converter15/1 -> [Relative_Vel]
  PS-Simulink Converter6/1 -> [Relative_wd]
  PS-Simulink Converter5/1 -> [Relative_quat]
  PS-Simulink Converter7/1 -> [Relative_w]
  Quaternions to Rotation Angles1/1 -> Radians to Degrees5/1
  Radians to Degrees5/1 -> Attitude:Rel,Iner/2
  From9/1 -> Scope12/1, Openning_Motion_Sequence2/1(b_flg)
  Openning_Motion_Sequence2/1(res) -> Gain1/1
  Quaternions to Rotation Angles2/1 -> Radians to Degrees6/1
  Radians to Degrees6/1 -> Attitude:Rel,Iner/1
  [Relative_quat] -> Quaternions to Rotation Angles2/1
  [S_Attitude_quat_Inertial] -> Quaternions to Rotation Angles1/1
  Openning_Motion_Sequence3/1(res) -> Gain5/1
  From19/1 -> Scope15/1, Openning_Motion_Sequence3/1(b_flg)
  [B_f_contact] -> Scope16/1, Openning_Motion_Sequence4/1(b_flg)
  Gain7/1 -> Down_ARM/1(J_cmd)
  Openning_Motion_Sequence4/2(mode) -> Down_ARM/2(Mode), Left_ARM/2(Mode), Right_ARM/2(Mode), Up_ARM/2(Mode)
  Gain8/1 -> Up_ARM/1(J_cmd)
  Gain9/1 -> Right_ARM/1(J_cmd)
  Openning_Motion_Sequence4/1(res) -> Left_ARM/1(J_cmd), Gain9/1, Gain8/1, Gain7/1
  [LEFT_ARM_Jt] -> Torq_Mea:LEFT,Right,Down,Up/1
  [Right_ARM_Jt] -> Torq_Mea:LEFT,Right,Down,Up/2
  [DOWN_ARM_Jt] -> Torq_Mea:LEFT,Right,Down,Up/3
  [Up_ARM_Jt] -> Torq_Mea:LEFT,Right,Down,Up/4
  [S_Attitude_quat_Inertial] -> Subsystem1/2(q)
  [Right_ARM_J] -> Radians to Degrees8/1
  [LEFT_ARM_J] -> Radians to Degrees7/1
  Radians to Degrees7/1 -> Display9/1, Joint_Angle_Mea:LEFT,Right,Down,Up/1
  Radians to Degrees8/1 -> Display10/1, Joint_Angle_Mea:LEFT,Right,Down,Up/2
  Radians to Degrees9/1 -> Display11/1, Joint_Angle_Mea:LEFT,Right,Down,Up/3
  Radians to Degrees10/1 -> Display12/1, Joint_Angle_Mea:LEFT,Right,Down,Up/4
  [LEFT_ARM_J] -> End_Position_Flg/1(L_J)
  [Right_ARM_J] -> End_Position_Flg/2(R_J)
  [Up_ARM_J] -> End_Position_Flg/3(U_J)
  [DOWN_ARM_J] -> End_Position_Flg/4(D_J)
  End_Position_Flg/1(res) -> [Pos_END_FLAG], Display13/1
  [DOWN_ARM_J] -> Radians to Degrees10/1
  [Up_ARM_J] -> Radians to Degrees9/1
  [Pos_END_FLAG] -> Openning_Motion_Sequence4/2(pos_end_flg)
  Right_ARM_Real_Simple_FK/2(ee_pose) -> Display16/1
  Right_ARM_Real_FK/2(ee_pose) -> Display14/1
  From33/1 -> Right_ARM_Real_FK/1(theta), Radians to Degrees11/1, Right_ARM_Real_Simple_FK/1(theta)
  From34/1 -> MATLAB Function4/1(u)
  MATLAB Function4/1(y) -> Display15/1
  Radians to Degrees11/1 -> Display17/1
  connections:
  Up_ARM/LConn4 -- Target/LConn1 -- Subsystem2/RConn2 -- Spatial Contact Force6/RConn1 -- Left_ARM/LConn4 -- Right_ARM/LConn4 -- Down_ARM/LConn4
  Transform Sensor2/LConn1 -- Brick Solid/LConn3 -- Down_ARM/LConn2 -- Up_ARM/LConn2 -- Right_ARM/LConn2 -- Left_ARM/LConn2 -- Transform Sensor5/RConn1 -- Transform Sensor1/RConn1
  6-DOF Joint2/LConn1 -- 6-DOF Joint1/LConn1 -- Solver Configuration/RConn1 -- World Frame/RConn1 -- Mechanism Configuration/RConn1
  6-DOF Joint1/RConn1 -- Transform Sensor2/RConn1 -- Target/RConn1
  Brick Solid/RConn1 -- 6-DOF Joint2/RConn1
  Brick Solid/LConn1 -- Left_ARM/LConn1
  Transform Sensor1/RConn3 -- PS-Simulink Converter2/LConn1
  Transform Sensor1/RConn2 -- PS-Simulink Converter1/LConn1
  Transform Sensor1/RConn4 -- PS-Simulink Converter3/LConn1
  Transform Sensor1/RConn5 -- PS-Simulink Converter4/LConn1
  Brick Solid/RConn2 -- Subsystem5/LConn1
  Transform Sensor5/RConn6 -- PS-Simulink Converter28/LConn1
  Transform Sensor5/RConn5 -- PS-Simulink Converter27/LConn1
  Transform Sensor5/RConn4 -- PS-Simulink Converter26/LConn1
  Transform Sensor5/RConn2 -- PS-Simulink Converter23/LConn1
  Transform Sensor5/RConn3 -- PS-Simulink Converter38/LConn1
  Right_ARM/LConn3 -- Left_ARM/LConn3 -- Brick Solid/LConn5 -- Spatial Contact Force6/LConn1 -- Up_ARM/LConn3 -- Down_ARM/LConn3
  Subsystem2/RConn1 -- Brick Solid/RConn3
  Transform Sensor2/RConn5 -- PS-Simulink Converter13/LConn1
  Transform Sensor2/RConn6 -- PS-Simulink Converter15/LConn1
  Transform Sensor2/RConn7 -- PS-Simulink Converter14/LConn1
  PS-Simulink Converter5/LConn1 -- Transform Sensor2/RConn2
  Transform Sensor2/RConn3 -- PS-Simulink Converter7/LConn1
  Transform Sensor2/RConn4 -- PS-Simulink Converter6/LConn1
  Brick Solid/LConn2 -- Right_ARM/LConn1
  Brick Solid/LConn4 -- Up_ARM/LConn1
  Down_ARM/LConn1 -- Brick Solid/RConn4
